simulink model "limbero_leg_control_DH"  (R2022a)
settings: Solver=ode45  StartTime=0.0  StopTime=8.00  RelTol=1e-3
undefined symbols (not defined in the file): a, a_contact, alpha, alpha_contact, d, d_contact, kpp, kpv, L, masses, masses_contact, offset, offset_contact, q_dotdot, qz, r_cm, r_cm_contact, t0, t_acc, T_lpf, t_tot, T_vel, Tc, Tiv
libraries: roblocks x4
settings Model: Creator=rubbe  LastModifiedBy=ale
settings ModelReferenceCC: EnableRefExpFcnMdlSchedulingChecks=off
settings RTWCC: Description=Generic Real-Time Target

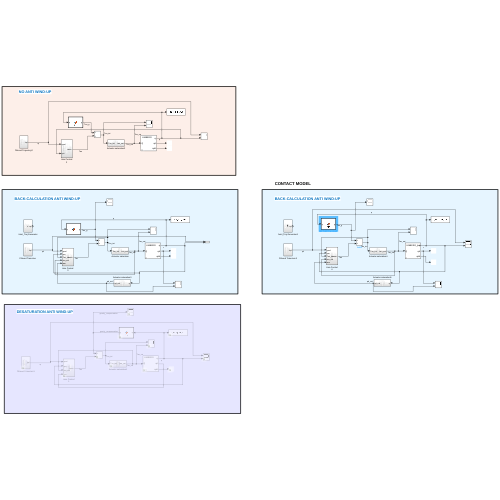
[thumbnail: Simulink's stored preview of the top-level diagram]
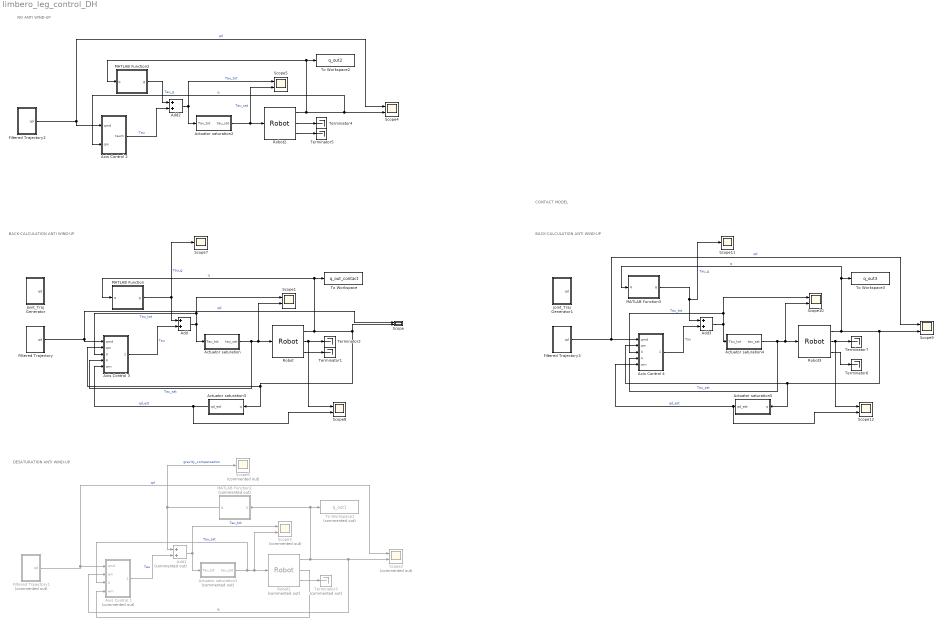
== system limbero_leg_control_DH ==
  note: CONTACT MODEL
  note: NO ANTI WIND-UP
  note: BACK-CALCULATION ANTI WIND-UP
  note: DESATURATION ANTI WIND-UP
  note: BACK-CALCULATION ANTI WIND-UP
  Actuator saturation : Subsystem
  Actuator saturation1 : Subsystem  Commented=on
  Actuator saturation2 : Subsystem
  Actuator saturation3 : Subsystem
  Actuator saturation4 : Subsystem
  Actuator saturation5 : Subsystem
  Add : Sum
  Add1 : Sum  Commented=on
  Add2 : Sum
  Add3 : Sum
  Axis Control 1 : Subsystem  Commented=on
  Axis Control 2 : Subsystem
  Axis Control 3 : Subsystem
  Axis Control 4 : Subsystem
  Filtered Trajectory : Subsystem
  Filtered Trajectory1 : Subsystem  Commented=on
  Filtered Trajectory2 : Subsystem
  Filtered Trajectory3 : Subsystem
  Joint_Traj Generator : Subsystem
  Joint_Traj Generator1 : Subsystem
  MATLAB Function : MATLAB Function  TreatAsAtomicUnit=on
  MATLAB Function1 : MATLAB Function  Commented=on  TreatAsAtomicUnit=on
  MATLAB Function2 : MATLAB Function  TreatAsAtomicUnit=on
  MATLAB Function3 : MATLAB Function  TreatAsAtomicUnit=on
  Robot : roblocks/Arm/Robot  robot=limbero  q0=qz'
  Robot1 : roblocks/Arm/Robot  Commented=on  robot=limbero  q0=qz'
  Robot2 : roblocks/Arm/Robot  robot=limbero  q0=qz'
  Robot3 : roblocks/Arm/Robot  robot=limbero_contact  q0=qz'
  Scope{,1,4..5,8..10,12} (8 alike) : Scope  NumInputPorts=2
  Scope11 : Scope
  Scope2 : Scope  Commented=on  NumInputPorts=2
  Scope3 : Scope  Commented=on  NumInputPorts=2
  Scope6 : Scope  Commented=on
  Scope7 : Scope
  Terminator{1..2,4..7} (6 alike) : Terminator
  Terminator3 : Terminator  Commented=on
  To Workspace : ToWorkspace  VariableName=q_out_contact  SaveFormat=Timeseries  SampleTime=-1
  To Workspace1 : ToWorkspace  Commented=on  VariableName=q_out1  SaveFormat=Timeseries  SampleTime=-1
  To Workspace2 : ToWorkspace  VariableName=q_out2  SaveFormat=Timeseries  SampleTime=-1
  To Workspace3 : ToWorkspace  VariableName=q_out3  SaveFormat=Timeseries  SampleTime=-1
  wires:
  Robot/3 -> Terminator1/1
  Robot/1 -> MATLAB Function/1(q), To Workspace/1, Axis Control 3/2(qm), Actuator saturation3/1(q), Scope/2  "q"
  MATLAB Function/1(g) -> Add/1, Scope7/1  "Tau_g"
  Filtered Trajectory/1(qd) -> Axis Control 3/1(qmd), Scope/1  "qd"
  Add/1 -> Axis Control 3/3(Tau_tot), Scope1/1, Actuator saturation/1(Tau_tot)  "Tau_tot"
  Actuator saturation/1(tau_sat) -> Axis Control 3/4(tau_sat), Robot/1, Scope1/2  "Tau_sat"
  Filtered Trajectory1/1(qd) -> Scope2/1, Axis Control 1/1(qmd)  "qd"
  Axis Control 1/1("taum ") -> Add1/2  "Tau"
  Actuator saturation1/1(tau_sat) -> Axis Control 1/3(tau_sat), Robot1/1, Scope3/2  "Tau_sat"
  Add1/1 -> Scope3/1, Actuator saturation1/1(Tau_tot)  "Tau_tot"
  Robot1/1 -> To Workspace1/1, MATLAB Function1/1(q), Scope2/2, Axis Control 1/2(qm)  "q"
  Robot1/3 -> Terminator3/1
  MATLAB Function1/1(g) -> Scope6/1, Add1/1  "gravity_compensation"
  Robot1/2 -> Axis Control 1/4(wm)
  Filtered Trajectory2/1(qd) -> Scope4/1, Axis Control 2/1(qmd)  "qd"
  Axis Control 2/1("taum ") -> Add2/2  "Tau"
  Actuator saturation2/1(tau_sat) -> Robot2/1, Scope5/2  "Tau_sat"
  Add2/1 -> Scope5/1, Actuator saturation2/1(Tau_tot)  "Tau_tot"
  Robot2/1 -> MATLAB Function2/1(q), To Workspace2/1, Scope4/2, Axis Control 2/2(qm)  "q"
  Robot2/3 -> Terminator5/1
  MATLAB Function2/1(g) -> Add2/1  "Tau_g"
  Robot2/2 -> Terminator4/1
  Axis Control 3/1("taum ") -> Add/2  "Tau"
  Robot/2 -> Scope8/1, Terminator2/1
  Actuator saturation3/1(qd_est) -> Scope8/2, Axis Control 3/5(wm)  "qd_est"
  Add3/1 -> Axis Control 4/3(Tau_tot), Scope10/1, Actuator saturation4/1(Tau_tot)  "Tau_tot"
  Filtered Trajectory3/1(qd) -> Axis Control 4/1(qmd), Scope9/1  "qd"
  Robot3/1 -> MATLAB Function3/1(q), To Workspace3/1, Axis Control 4/2(qm), Actuator saturation5/1(q), Scope9/2  "q"
  MATLAB Function3/1(g) -> Scope11/1, Add3/1  "Tau_g"
  Robot3/3 -> Terminator6/1
  Robot3/2 -> Scope12/1, Terminator7/1
  Actuator saturation4/1(tau_sat) -> Axis Control 4/4(tau_sat), Robot3/1, Scope10/2  "Tau_sat"
  Actuator saturation5/1(qd_est) -> Scope12/2, Axis Control 4/5(wm)  "qd_est"
  Axis Control 4/1("taum ") -> Add3/2  "Tau"

== system limbero_leg_control_DH/Actuator saturation ==
  Tau_tot : Inport
  Demux : Demux  Outputs=7
  Mux : Mux  Inputs=7
  Saturation : Saturate  UpperLimit=20.0  LowerLimit=-20.0
  Saturation1 : Saturate  UpperLimit=20.0  LowerLimit=-20.0
  Saturation2 : Saturate  UpperLimit=12.0  LowerLimit=-12.0
  Saturation3 : Saturate  UpperLimit=14.0  LowerLimit=-14.0
  Saturation4 : Saturate  UpperLimit=12.0  LowerLimit=-12.0
  Saturation5 : Saturate  UpperLimit=14.0  LowerLimit=-14.0
  Saturation6 : Saturate  UpperLimit=12.0  LowerLimit=-12.0
  tau_sat : Outport
  wires:
  Saturation6/1 -> Mux/7
  Mux/1 -> tau_sat/1
  Saturation3/1 -> Mux/4
  Tau_tot/1 -> Demux/1
  Demux/4 -> Saturation3/1
  Demux/7 -> Saturation6/1
  Saturation4/1 -> Mux/5
  Saturation1/1 -> Mux/2
  Demux/3 -> Saturation2/1
  Demux/1 -> Saturation/1
  Demux/5 -> Saturation4/1
  Demux/6 -> Saturation5/1
  Demux/2 -> Saturation1/1
  Saturation/1 -> Mux/1
  Saturation5/1 -> Mux/6
  Saturation2/1 -> Mux/3

== system limbero_leg_control_DH/Actuator saturation1 ==
  Tau_tot : Inport
  Demux : Demux  Outputs=7
  Mux : Mux  Inputs=7
  Saturation : Saturate  UpperLimit=20.0  LowerLimit=-20.0
  Saturation1 : Saturate  UpperLimit=20.0  LowerLimit=-20.0
  Saturation2 : Saturate  UpperLimit=12.0  LowerLimit=-12.0
  Saturation3 : Saturate  UpperLimit=14.0  LowerLimit=-14.0
  Saturation4 : Saturate  UpperLimit=12.0  LowerLimit=-12.0
  Saturation5 : Saturate  UpperLimit=14.0  LowerLimit=-14.0
  Saturation6 : Saturate  UpperLimit=12.0  LowerLimit=-12.0
  tau_sat : Outport
  wires:
  Saturation6/1 -> Mux/7
  Mux/1 -> tau_sat/1
  Saturation3/1 -> Mux/4
  Tau_tot/1 -> Demux/1
  Demux/4 -> Saturation3/1
  Demux/7 -> Saturation6/1
  Saturation4/1 -> Mux/5
  Saturation1/1 -> Mux/2
  Demux/3 -> Saturation2/1
  Demux/1 -> Saturation/1
  Demux/5 -> Saturation4/1
  Demux/6 -> Saturation5/1
  Demux/2 -> Saturation1/1
  Saturation/1 -> Mux/1
  Saturation5/1 -> Mux/6
  Saturation2/1 -> Mux/3

== system limbero_leg_control_DH/Actuator saturation2 ==
  Tau_tot : Inport
  Demux : Demux  Outputs=7
  Mux : Mux  Inputs=7
  Saturation : Saturate  UpperLimit=20.0  LowerLimit=-20.0
  Saturation1 : Saturate  UpperLimit=20.0  LowerLimit=-20.0
  Saturation2 : Saturate  UpperLimit=12.0  LowerLimit=-12.0
  Saturation3 : Saturate  UpperLimit=14.0  LowerLimit=-14.0
  Saturation4 : Saturate  UpperLimit=12.0  LowerLimit=-12.0
  Saturation5 : Saturate  UpperLimit=14.0  LowerLimit=-14.0
  Saturation6 : Saturate  UpperLimit=12.0  LowerLimit=-12.0
  tau_sat : Outport
  wires:
  Saturation6/1 -> Mux/7
  Mux/1 -> tau_sat/1
  Saturation3/1 -> Mux/4
  Tau_tot/1 -> Demux/1
  Demux/4 -> Saturation3/1
  Demux/7 -> Saturation6/1
  Saturation4/1 -> Mux/5
  Saturation1/1 -> Mux/2
  Demux/3 -> Saturation2/1
  Demux/1 -> Saturation/1
  Demux/5 -> Saturation4/1
  Demux/6 -> Saturation5/1
  Demux/2 -> Saturation1/1
  Saturation/1 -> Mux/1
  Saturation5/1 -> Mux/6
  Saturation2/1 -> Mux/3

== system limbero_leg_control_DH/Actuator saturation3 ==
  q : Inport
  Demux : Demux  Outputs=7
  Mux : Mux  Inputs=7
  Transfer Fcn{,1..6} (7 alike) : TransferFcn  Numerator=[1 0]  Denominator=[T_vel 1]
  qd_est : Outport
  wires:
  Mux/1 -> qd_est/1
  q/1 -> Demux/1
  Demux/4 -> Transfer Fcn3/1
  Demux/7 -> Transfer Fcn6/1
  Transfer Fcn1/1 -> Mux/2
  Demux/3 -> Transfer Fcn2/1
  Demux/1 -> Transfer Fcn/1
  Demux/5 -> Transfer Fcn4/1
  Demux/6 -> Transfer Fcn5/1
  Demux/2 -> Transfer Fcn1/1
  Transfer Fcn/1 -> Mux/1
  Transfer Fcn6/1 -> Mux/7
  Transfer Fcn5/1 -> Mux/6
  Transfer Fcn4/1 -> Mux/5
  Transfer Fcn3/1 -> Mux/4
  Transfer Fcn2/1 -> Mux/3

== system limbero_leg_control_DH/Actuator saturation4 ==
  Tau_tot : Inport
  Demux : Demux  Outputs=7
  Mux : Mux  Inputs=7
  Saturation : Saturate  UpperLimit=20.0  LowerLimit=-20.0
  Saturation1 : Saturate  UpperLimit=20.0  LowerLimit=-20.0
  Saturation2 : Saturate  UpperLimit=12.0  LowerLimit=-12.0
  Saturation3 : Saturate  UpperLimit=14.0  LowerLimit=-14.0
  Saturation4 : Saturate  UpperLimit=12.0  LowerLimit=-12.0
  Saturation5 : Saturate  UpperLimit=14.0  LowerLimit=-14.0
  Saturation6 : Saturate  UpperLimit=12.0  LowerLimit=-12.0
  tau_sat : Outport
  wires:
  Saturation6/1 -> Mux/7
  Mux/1 -> tau_sat/1
  Saturation3/1 -> Mux/4
  Tau_tot/1 -> Demux/1
  Demux/4 -> Saturation3/1
  Demux/7 -> Saturation6/1
  Saturation4/1 -> Mux/5
  Saturation1/1 -> Mux/2
  Demux/3 -> Saturation2/1
  Demux/1 -> Saturation/1
  Demux/5 -> Saturation4/1
  Demux/6 -> Saturation5/1
  Demux/2 -> Saturation1/1
  Saturation/1 -> Mux/1
  Saturation5/1 -> Mux/6
  Saturation2/1 -> Mux/3

== system limbero_leg_control_DH/Actuator saturation5 ==
  q : Inport
  Demux : Demux  Outputs=7
  Mux : Mux  Inputs=7
  Transfer Fcn{,1..6} (7 alike) : TransferFcn  Numerator=[1 0]  Denominator=[T_vel 1]
  qd_est : Outport
  wires:
  Mux/1 -> qd_est/1
  q/1 -> Demux/1
  Demux/4 -> Transfer Fcn3/1
  Demux/7 -> Transfer Fcn6/1
  Transfer Fcn1/1 -> Mux/2
  Demux/3 -> Transfer Fcn2/1
  Demux/1 -> Transfer Fcn/1
  Demux/5 -> Transfer Fcn4/1
  Demux/6 -> Transfer Fcn5/1
  Demux/2 -> Transfer Fcn1/1
  Transfer Fcn/1 -> Mux/1
  Transfer Fcn6/1 -> Mux/7
  Transfer Fcn5/1 -> Mux/6
  Transfer Fcn4/1 -> Mux/5
  Transfer Fcn3/1 -> Mux/4
  Transfer Fcn2/1 -> Mux/3

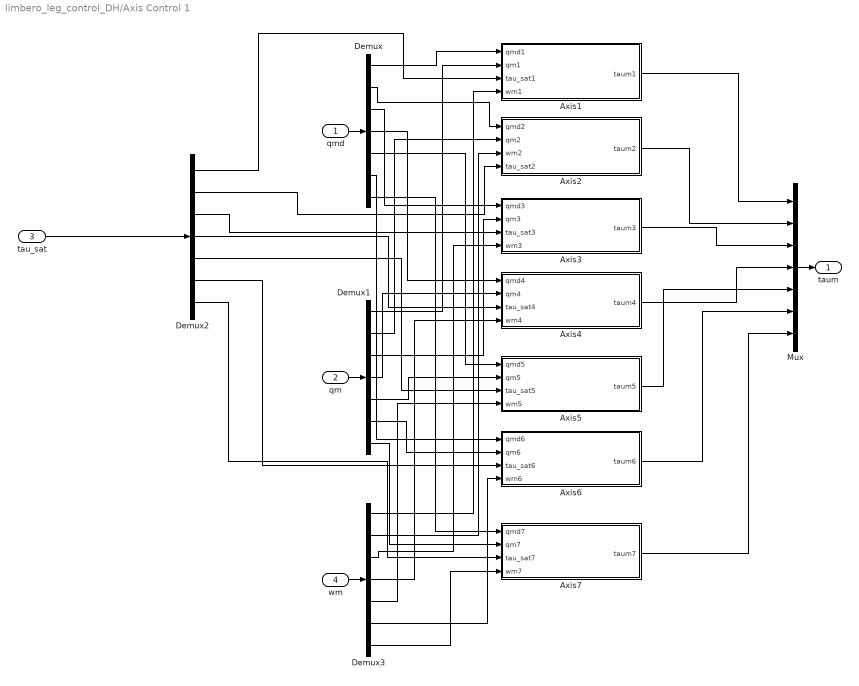
== system limbero_leg_control_DH/Axis Control 1 ==
  qmd : Inport
  qm : Inport  Port=2
  tau_sat : Inport  Port=3
  wm : Inport  Port=4
  "Axis1 " : Subsystem
  "Axis2 " : Subsystem
  "Axis3 " : Subsystem
  "Axis4 " : Subsystem
  "Axis5 " : Subsystem
  "Axis6 " : Subsystem
  "Axis7 " : Subsystem
  Demux{,1..3} (4 alike) : Demux  Outputs=7
  Mux : Mux  Inputs=7
  "taum " : Outport  VectorParamsAs1DForOutWhenUnconnected=off
  wires:
  "Axis5 "/1(taum5) -> Mux/5
  Demux1/1 -> "Axis1 "/2(qm1)
  Demux1/3 -> "Axis3 "/2(qm3)
  Demux/1 -> "Axis1 "/1(qmd1)
  "Axis4 "/1(taum4) -> Mux/4
  "Axis3 "/1(taum3) -> Mux/3
  "Axis6 "/1(taum6) -> Mux/6
  "Axis1 "/1(taum1) -> Mux/1
  Mux/1 -> "taum "/1
  Demux/2 -> "Axis2 "/1(qmd2)
  Demux/4 -> "Axis4 "/1(qmd4)
  Demux/3 -> "Axis3 "/1(qmd3)
  Demux/6 -> "Axis6 "/1(qmd6)
  Demux/5 -> "Axis5 "/1(qmd5)
  Demux1/4 -> "Axis4 "/2(qm4)
  Demux1/6 -> "Axis6 "/2(qm6)
  Demux1/5 -> "Axis5 "/2(qm5)
  Demux1/2 -> "Axis2 "/2(qm2)
  qm/1 -> Demux1/1
  qmd/1 -> Demux/1
  Demux1/7 -> "Axis7 "/2(qm7)
  Demux/7 -> "Axis7 "/1(qmd7)
  "Axis7 "/1(taum7) -> Mux/7
  Demux2/7 -> "Axis7 "/3(tau_sat7)
  tau_sat/1 -> Demux2/1
  Demux2/6 -> "Axis6 "/3(tau_sat6)
  Demux2/5 -> "Axis5 "/3(tau_sat5)
  Demux2/4 -> "Axis4 "/3(tau_sat4)
  Demux2/3 -> "Axis3 "/3(tau_sat3)
  Demux2/1 -> "Axis1 "/3(tau_sat1)
  wm/1 -> Demux3/1
  Demux3/1 -> "Axis1 "/4(wm1)
  Demux3/2 -> "Axis2 "/3(wm2)
  Demux3/3 -> "Axis3 "/4(wm3)
  Demux3/4 -> "Axis4 "/4(wm4)
  Demux3/5 -> "Axis5 "/4(wm5)
  Demux3/6 -> "Axis6 "/4(wm6)
  Demux3/7 -> "Axis7 "/4(wm7)
  Demux2/2 -> "Axis2 "/4(tau_sat2)
  "Axis2 "/1(taum2) -> Mux/2

== system limbero_leg_control_DH/Axis Control 2 ==
  qmd : Inport
  qm : Inport  Port=2
  "Axis1 " : Subsystem
  "Axis2 " : Subsystem
  "Axis3 " : Subsystem
  "Axis4 " : Subsystem
  "Axis5 " : Subsystem
  "Axis6 " : Subsystem
  "Axis7 " : Subsystem
  Demux : Demux  Outputs=7
  Demux1 : Demux  Outputs=7
  Mux : Mux  Inputs=7
  "taum " : Outport  VectorParamsAs1DForOutWhenUnconnected=off
  wires:
  "Axis5 "/1(taum5) -> Mux/5
  Demux1/1 -> "Axis1 "/2(qm1)
  "Axis2 "/1(taum2) -> Mux/2
  Demux1/3 -> "Axis3 "/2(qm3)
  Demux/1 -> "Axis1 "/1(qmd1)
  "Axis4 "/1(taum4) -> Mux/4
  "Axis3 "/1(taum3) -> Mux/3
  "Axis6 "/1(taum6) -> Mux/6
  "Axis1 "/1(taum1) -> Mux/1
  Mux/1 -> "taum "/1
  Demux/2 -> "Axis2 "/1(qmd2)
  Demux/4 -> "Axis4 "/1(qmd4)
  Demux/3 -> "Axis3 "/1(qmd3)
  Demux/6 -> "Axis6 "/1(qmd6)
  Demux/5 -> "Axis5 "/1(qmd5)
  Demux1/4 -> "Axis4 "/2(qm4)
  Demux1/6 -> "Axis6 "/2(qm6)
  Demux1/5 -> "Axis5 "/2(qm5)
  Demux1/2 -> "Axis2 "/2(qm2)
  qm/1 -> Demux1/1
  qmd/1 -> Demux/1
  Demux1/7 -> "Axis7 "/2(qm7)
  Demux/7 -> "Axis7 "/1(qmd7)
  "Axis7 "/1(taum7) -> Mux/7

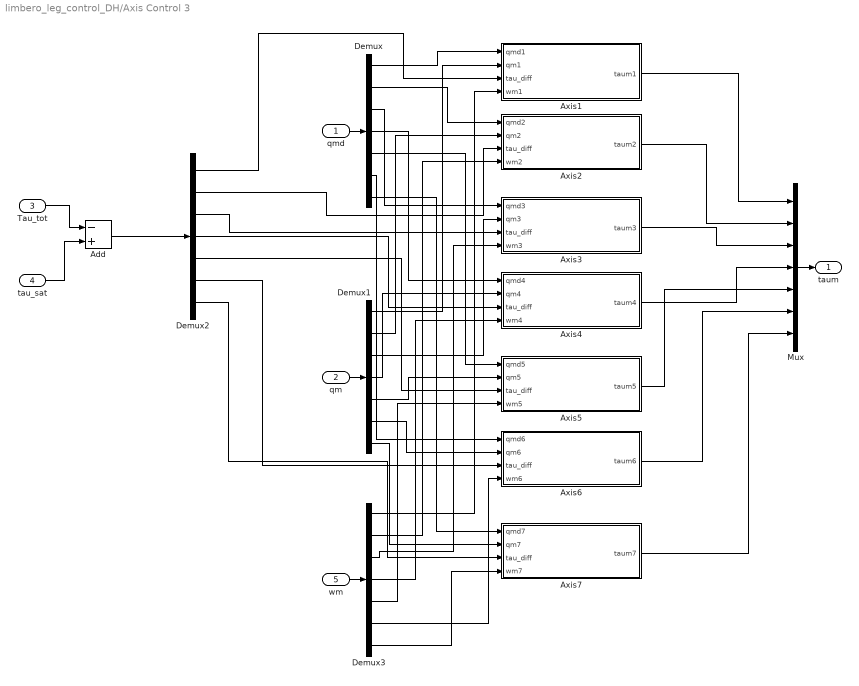
== system limbero_leg_control_DH/Axis Control 3 ==
  qmd : Inport
  qm : Inport  Port=2
  Tau_tot : Inport  Port=3
  tau_sat : Inport  Port=4
  wm : Inport  Port=5
  Add : Sum  Inputs=-+
  "Axis1 " : Subsystem
  "Axis2 " : Subsystem
  "Axis3 " : Subsystem
  "Axis4 " : Subsystem
  "Axis5 " : Subsystem
  "Axis6 " : Subsystem
  "Axis7 " : Subsystem
  Demux{,1..3} (4 alike) : Demux  Outputs=7
  Mux : Mux  Inputs=7
  "taum " : Outport  VectorParamsAs1DForOutWhenUnconnected=off
  wires:
  "Axis5 "/1(taum5) -> Mux/5
  Demux1/1 -> "Axis1 "/2(qm1)
  "Axis2 "/1(taum2) -> Mux/2
  Demux1/3 -> "Axis3 "/2(qm3)
  Demux/1 -> "Axis1 "/1(qmd1)
  "Axis4 "/1(taum4) -> Mux/4
  "Axis3 "/1(taum3) -> Mux/3
  "Axis6 "/1(taum6) -> Mux/6
  "Axis1 "/1(taum1) -> Mux/1
  Mux/1 -> "taum "/1
  Demux/2 -> "Axis2 "/1(qmd2)
  Demux/4 -> "Axis4 "/1(qmd4)
  Demux/3 -> "Axis3 "/1(qmd3)
  Demux/6 -> "Axis6 "/1(qmd6)
  Demux/5 -> "Axis5 "/1(qmd5)
  Demux1/4 -> "Axis4 "/2(qm4)
  Demux1/6 -> "Axis6 "/2(qm6)
  Demux1/5 -> "Axis5 "/2(qm5)
  Demux1/2 -> "Axis2 "/2(qm2)
  qm/1 -> Demux1/1
  qmd/1 -> Demux/1
  Demux1/7 -> "Axis7 "/2(qm7)
  Demux/7 -> "Axis7 "/1(qmd7)
  "Axis7 "/1(taum7) -> Mux/7
  Tau_tot/1 -> Add/1
  tau_sat/1 -> Add/2
  Demux2/7 -> "Axis7 "/3(tau_diff)
  Add/1 -> Demux2/1
  Demux2/6 -> "Axis6 "/3(tau_diff)
  Demux2/5 -> "Axis5 "/3(tau_diff)
  Demux2/4 -> "Axis4 "/3(tau_diff)
  Demux2/3 -> "Axis3 "/3(tau_diff)
  Demux2/2 -> "Axis2 "/3(tau_diff)
  Demux2/1 -> "Axis1 "/3(tau_diff)
  wm/1 -> Demux3/1
  Demux3/1 -> "Axis1 "/4(wm1)
  Demux3/2 -> "Axis2 "/4(wm2)
  Demux3/3 -> "Axis3 "/4(wm3)
  Demux3/4 -> "Axis4 "/4(wm4)
  Demux3/5 -> "Axis5 "/4(wm5)
  Demux3/6 -> "Axis6 "/4(wm6)
  Demux3/7 -> "Axis7 "/4(wm7)

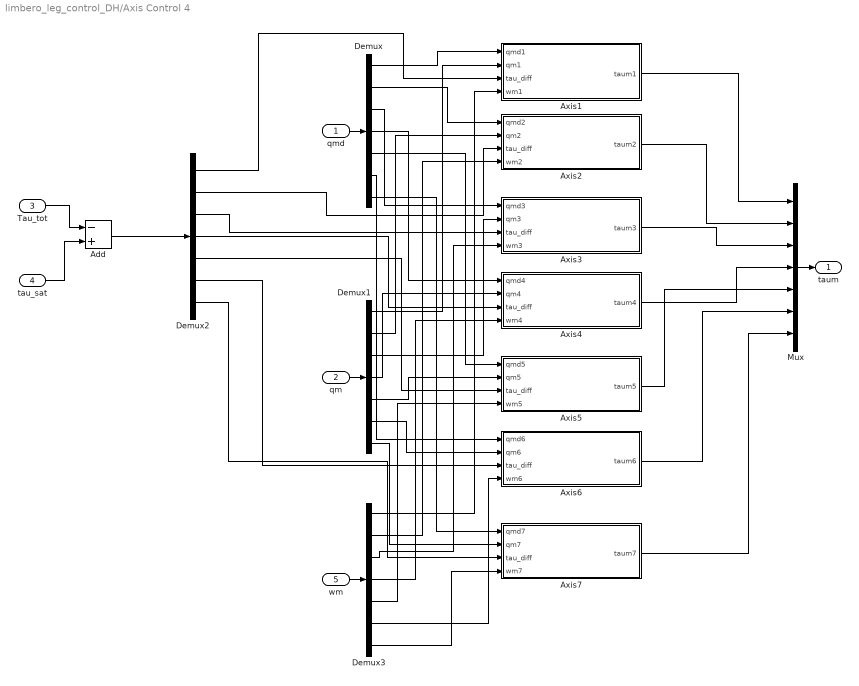
== system limbero_leg_control_DH/Axis Control 4 ==
  qmd : Inport
  qm : Inport  Port=2
  Tau_tot : Inport  Port=3
  tau_sat : Inport  Port=4
  wm : Inport  Port=5
  Add : Sum  Inputs=-+
  "Axis1 " : Subsystem
  "Axis2 " : Subsystem
  "Axis3 " : Subsystem
  "Axis4 " : Subsystem
  "Axis5 " : Subsystem
  "Axis6 " : Subsystem
  "Axis7 " : Subsystem
  Demux{,1..3} (4 alike) : Demux  Outputs=7
  Mux : Mux  Inputs=7
  "taum " : Outport  VectorParamsAs1DForOutWhenUnconnected=off
  wires:
  "Axis5 "/1(taum5) -> Mux/5
  Demux1/1 -> "Axis1 "/2(qm1)
  "Axis2 "/1(taum2) -> Mux/2
  Demux1/3 -> "Axis3 "/2(qm3)
  Demux/1 -> "Axis1 "/1(qmd1)
  "Axis4 "/1(taum4) -> Mux/4
  "Axis3 "/1(taum3) -> Mux/3
  "Axis6 "/1(taum6) -> Mux/6
  "Axis1 "/1(taum1) -> Mux/1
  Mux/1 -> "taum "/1
  Demux/2 -> "Axis2 "/1(qmd2)
  Demux/4 -> "Axis4 "/1(qmd4)
  Demux/3 -> "Axis3 "/1(qmd3)
  Demux/6 -> "Axis6 "/1(qmd6)
  Demux/5 -> "Axis5 "/1(qmd5)
  Demux1/4 -> "Axis4 "/2(qm4)
  Demux1/6 -> "Axis6 "/2(qm6)
  Demux1/5 -> "Axis5 "/2(qm5)
  Demux1/2 -> "Axis2 "/2(qm2)
  qm/1 -> Demux1/1
  qmd/1 -> Demux/1
  Demux1/7 -> "Axis7 "/2(qm7)
  Demux/7 -> "Axis7 "/1(qmd7)
  "Axis7 "/1(taum7) -> Mux/7
  Tau_tot/1 -> Add/1
  tau_sat/1 -> Add/2
  Demux2/7 -> "Axis7 "/3(tau_diff)
  Add/1 -> Demux2/1
  Demux2/6 -> "Axis6 "/3(tau_diff)
  Demux2/5 -> "Axis5 "/3(tau_diff)
  Demux2/4 -> "Axis4 "/3(tau_diff)
  Demux2/3 -> "Axis3 "/3(tau_diff)
  Demux2/2 -> "Axis2 "/3(tau_diff)
  Demux2/1 -> "Axis1 "/3(tau_diff)
  wm/1 -> Demux3/1
  Demux3/1 -> "Axis1 "/4(wm1)
  Demux3/2 -> "Axis2 "/4(wm2)
  Demux3/3 -> "Axis3 "/4(wm3)
  Demux3/4 -> "Axis4 "/4(wm4)
  Demux3/5 -> "Axis5 "/4(wm5)
  Demux3/6 -> "Axis6 "/4(wm6)
  Demux3/7 -> "Axis7 "/4(wm7)

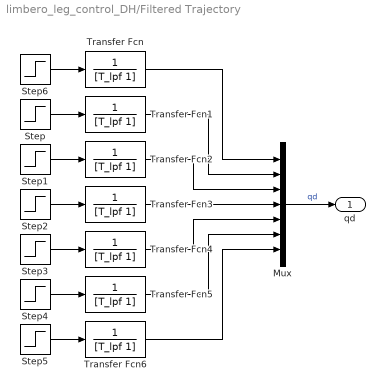
== system limbero_leg_control_DH/Filtered Trajectory ==
  Mux : Mux  Inputs=7
  Step{,1..2,5..6} (5 alike) : Step  Time=0  After=0  SampleTime=0
  Step3 : Step  After=-pi/6  SampleTime=0
  Step4 : Step  Time=2  After=-pi/8  SampleTime=0
  Transfer Fcn{,1..6} (7 alike) : TransferFcn  Denominator=[T_lpf 1]
  qd : Outport
  wires:
  Step3/1 -> Transfer Fcn4/1
  Step1/1 -> Transfer Fcn2/1
  Step4/1 -> Transfer Fcn5/1
  Transfer Fcn/1 -> Mux/1
  Transfer Fcn6/1 -> Mux/7
  Transfer Fcn3/1 -> Mux/4
  Transfer Fcn5/1 -> Mux/6
  Step2/1 -> Transfer Fcn3/1
  Step/1 -> Transfer Fcn1/1
  Step6/1 -> Transfer Fcn/1
  Transfer Fcn2/1 -> Mux/3
  Transfer Fcn4/1 -> Mux/5
  Transfer Fcn1/1 -> Mux/2
  Mux/1 -> qd/1  "qd"
  Step5/1 -> Transfer Fcn6/1

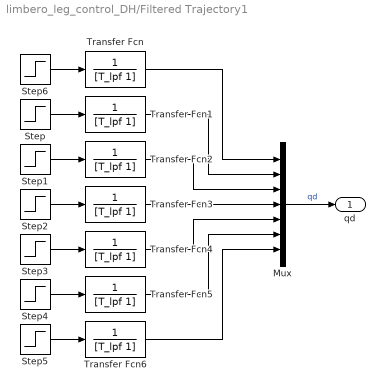
== system limbero_leg_control_DH/Filtered Trajectory1 ==
  Mux : Mux  Inputs=7
  Step : Step  After=-pi/6  SampleTime=0
  Step1 : Step  After=pi/2  SampleTime=0
  Step2 : Step  After=0  SampleTime=0
  Step3 : Step  Time=0  After=0  SampleTime=0
  Step4 : Step  Time=0  After=0  SampleTime=0
  Step5 : Step  Time=0  After=0  SampleTime=0
  Step6 : Step  Time=0.5  After=pi/4  SampleTime=0
  Transfer Fcn{,1..6} (7 alike) : TransferFcn  Denominator=[T_lpf 1]
  qd : Outport
  wires:
  Step3/1 -> Transfer Fcn4/1
  Step1/1 -> Transfer Fcn2/1
  Step4/1 -> Transfer Fcn5/1
  Transfer Fcn/1 -> Mux/1
  Transfer Fcn6/1 -> Mux/7
  Transfer Fcn3/1 -> Mux/4
  Transfer Fcn5/1 -> Mux/6
  Step2/1 -> Transfer Fcn3/1
  Step/1 -> Transfer Fcn1/1
  Step6/1 -> Transfer Fcn/1
  Transfer Fcn2/1 -> Mux/3
  Transfer Fcn4/1 -> Mux/5
  Transfer Fcn1/1 -> Mux/2
  Mux/1 -> qd/1  "qd"
  Step5/1 -> Transfer Fcn6/1

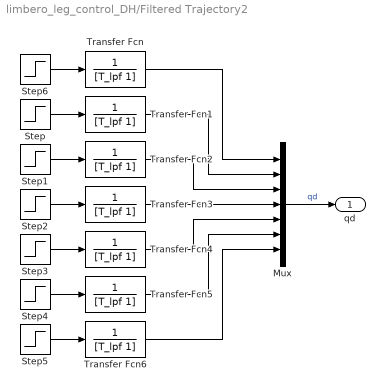
== system limbero_leg_control_DH/Filtered Trajectory2 ==
  Mux : Mux  Inputs=7
  Step : Step  After=-pi/6  SampleTime=0
  Step1 : Step  After=pi/2  SampleTime=0
  Step2 : Step  After=0  SampleTime=0
  Step3 : Step  Time=0  After=0  SampleTime=0
  Step4 : Step  Time=0  After=0  SampleTime=0
  Step5 : Step  Time=0  After=0  SampleTime=0
  Step6 : Step  Time=0.5  After=pi/4  SampleTime=0
  Transfer Fcn{,1..6} (7 alike) : TransferFcn  Denominator=[T_lpf 1]
  qd : Outport
  wires:
  Step3/1 -> Transfer Fcn4/1
  Step1/1 -> Transfer Fcn2/1
  Step4/1 -> Transfer Fcn5/1
  Transfer Fcn/1 -> Mux/1
  Transfer Fcn6/1 -> Mux/7
  Transfer Fcn3/1 -> Mux/4
  Transfer Fcn5/1 -> Mux/6
  Step2/1 -> Transfer Fcn3/1
  Step/1 -> Transfer Fcn1/1
  Step6/1 -> Transfer Fcn/1
  Transfer Fcn2/1 -> Mux/3
  Transfer Fcn4/1 -> Mux/5
  Transfer Fcn1/1 -> Mux/2
  Mux/1 -> qd/1  "qd"
  Step5/1 -> Transfer Fcn6/1

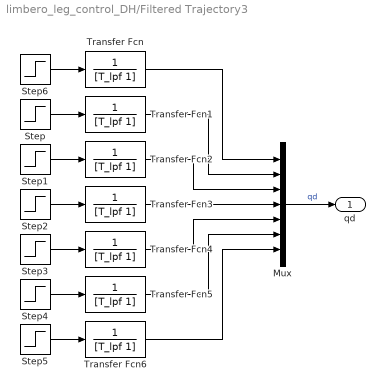
== system limbero_leg_control_DH/Filtered Trajectory3 ==
  Mux : Mux  Inputs=7
  Step : Step  After=-pi/6  SampleTime=0
  Step1 : Step  After=pi/2  SampleTime=0
  Step2 : Step  After=0  SampleTime=0
  Step3 : Step  Time=0  After=0  SampleTime=0
  Step4 : Step  Time=0  After=0  SampleTime=0
  Step5 : Step  Time=0  After=0  SampleTime=0
  Step6 : Step  Time=0.5  After=pi/4  SampleTime=0
  Transfer Fcn{,1..6} (7 alike) : TransferFcn  Denominator=[T_lpf 1]
  qd : Outport
  wires:
  Step3/1 -> Transfer Fcn4/1
  Step1/1 -> Transfer Fcn2/1
  Step4/1 -> Transfer Fcn5/1
  Transfer Fcn/1 -> Mux/1
  Transfer Fcn6/1 -> Mux/7
  Transfer Fcn3/1 -> Mux/4
  Transfer Fcn5/1 -> Mux/6
  Step2/1 -> Transfer Fcn3/1
  Step/1 -> Transfer Fcn1/1
  Step6/1 -> Transfer Fcn/1
  Transfer Fcn2/1 -> Mux/3
  Transfer Fcn4/1 -> Mux/5
  Transfer Fcn1/1 -> Mux/2
  Mux/1 -> qd/1  "qd"
  Step5/1 -> Transfer Fcn6/1

== system limbero_leg_control_DH/Joint_Traj Generator ==
  Constant : Constant  Value=0
  Mux : Mux  Inputs=7
  Subsystem : Subsystem
  Subsystem1 : Subsystem
  qd : Outport
  wires:
  Subsystem1/1(C2F) -> Mux/3
  Constant/1 -> Mux/7, Mux/6, Mux/5, Mux/4, Mux/1
  Subsystem/1(B2C) -> Mux/2
  Mux/1 -> qd/1

== system limbero_leg_control_DH/Joint_Traj Generator1 ==
  Constant : Constant  Value=0
  Mux : Mux  Inputs=7
  Subsystem : Subsystem
  Subsystem1 : Subsystem
  qd : Outport
  wires:
  Subsystem1/1(C2F) -> Mux/3
  Constant/1 -> Mux/7, Mux/6, Mux/5, Mux/4, Mux/1
  Subsystem/1(B2C) -> Mux/2
  Mux/1 -> qd/1

== system limbero_leg_control_DH/Axis Control 1/Axis1  ==
  qmd1 : Inport
  qm1 : Inport  Port=2
  tau_sat1 : Inport  Port=3
  wm1 : Inport  Port=4
  Add : Sum  Inputs=++-
  Add1 : Sum
  "Derivator qmd1 " : Derivative  CoefficientInTFapproximation=1/260
  Prop 1 : Gain  Gain=kpp
  Sum : Sum  Inputs=|+-
  Transfer Fcn4 : TransferFcn  Numerator=[kpv(1)*Tiv kpv(1)]  Denominator=[Tiv L]
  Transfer Fcn5 : TransferFcn  Numerator=[L]  Denominator=[Tiv L]
  taum1 : Outport  VectorParamsAs1DForOutWhenUnconnected=off
  wires:
  "Derivator qmd1 "/1 -> Add/1
  Sum/1 -> Prop 1/1
  qm1/1 -> Sum/2
  Prop 1/1 -> Add/2
  qmd1/1 -> "Derivator qmd1 "/1, Sum/1
  Add1/1 -> taum1/1
  wm1/1 -> Add/3  "wm1"
  Add/1 -> Transfer Fcn4/1
  Transfer Fcn4/1 -> Add1/1
  tau_sat1/1 -> Transfer Fcn5/1
  Transfer Fcn5/1 -> Add1/2  "anti_wind_up"

== system limbero_leg_control_DH/Axis Control 1/Axis2  ==
  qmd2 : Inport
  qm2 : Inport  Port=2
  wm2 : Inport  Port=3
  tau_sat2 : Inport  Port=4
  Add : Sum  Inputs=++-
  Add1 : Sum
  Derivator qmd2 : Derivative  CoefficientInTFapproximation=1/260
  Prop 2 : Gain  Gain=kpp
  Scope : Scope
  Scope1 : Scope
  Sum : Sum  Inputs=|+-
  Transfer Fcn4 : TransferFcn  Numerator=[kpv(2)*Tiv kpv(2)]  Denominator=[Tiv L]
  Transfer Fcn5 : TransferFcn  Numerator=[L]  Denominator=[Tiv L]
  taum2 : Outport  VectorParamsAs1DForOutWhenUnconnected=off
  wires:
  Derivator qmd2/1 -> Add/1
  Sum/1 -> Prop 2/1
  qm2/1 -> Sum/2
  Prop 2/1 -> Add/2
  qmd2/1 -> Derivator qmd2/1, Sum/1
  wm2/1 -> Add/3
  tau_sat2/1 -> Transfer Fcn5/1
  Transfer Fcn4/1 -> Add1/1
  Add/1 -> Scope/1, Transfer Fcn4/1  "e_w"
  Transfer Fcn5/1 -> Scope1/1, Add1/2  "anti_wind_up"
  Add1/1 -> taum2/1

== system limbero_leg_control_DH/Axis Control 1/Axis3  ==
  qmd3 : Inport
  qm3 : Inport  Port=2
  tau_sat3 : Inport  Port=3
  wm3 : Inport  Port=4
  Add : Sum  Inputs=++-
  Add1 : Sum
  Derivator qmd3 : Derivative  CoefficientInTFapproximation=1/260
  Prop 3 : Gain  Gain=kpp
  Sum : Sum  Inputs=|+-
  Transfer Fcn4 : TransferFcn  Numerator=[kpv(3)*Tiv kpv(3)]  Denominator=[Tiv L]
  Transfer Fcn5 : TransferFcn  Numerator=[L]  Denominator=[Tiv L]
  taum3 : Outport  VectorParamsAs1DForOutWhenUnconnected=off
  wires:
  Derivator qmd3/1 -> Add/1
  wm3/1 -> Add/3
  Sum/1 -> Prop 3/1
  qm3/1 -> Sum/2
  Prop 3/1 -> Add/2
  qmd3/1 -> Derivator qmd3/1, Sum/1
  Add1/1 -> taum3/1
  Transfer Fcn5/1 -> Add1/2  "anti_wind_up"
  Transfer Fcn4/1 -> Add1/1
  Add/1 -> Transfer Fcn4/1
  tau_sat3/1 -> Transfer Fcn5/1

== system limbero_leg_control_DH/Axis Control 1/Axis4  ==
  qmd4 : Inport
  qm4 : Inport  Port=2
  tau_sat4 : Inport  Port=3
  wm4 : Inport  Port=4
  Add : Sum  Inputs=++-
  Add1 : Sum
  Derivator qmd4 : Derivative  CoefficientInTFapproximation=1/700
  Prop 4 : Gain  Gain=kpp
  Sum : Sum  Inputs=|+-
  Transfer Fcn4 : TransferFcn  Numerator=[kpv(4)*Tiv kpv(4)]  Denominator=[Tiv L]
  Transfer Fcn5 : TransferFcn  Numerator=[L]  Denominator=[Tiv L]
  taum4 : Outport  VectorParamsAs1DForOutWhenUnconnected=off
  wires:
  Derivator qmd4/1 -> Add/1
  wm4/1 -> Add/3
  Sum/1 -> Prop 4/1
  qm4/1 -> Sum/2
  Prop 4/1 -> Add/2
  qmd4/1 -> Derivator qmd4/1, Sum/1
  tau_sat4/1 -> Transfer Fcn5/1
  Transfer Fcn5/1 -> Add1/2  "anti_wind_up"
  Transfer Fcn4/1 -> Add1/1
  Add/1 -> Transfer Fcn4/1
  Add1/1 -> taum4/1

== system limbero_leg_control_DH/Axis Control 1/Axis5  ==
  qmd5 : Inport
  qm5 : Inport  Port=2
  tau_sat5 : Inport  Port=3
  wm5 : Inport  Port=4
  Add : Sum  Inputs=++-
  Add1 : Sum
  Derivator qmd5 : Derivative  CoefficientInTFapproximation=1/700
  Prop 5 : Gain  Gain=kpp
  Sum : Sum  Inputs=|+-
  Transfer Fcn4 : TransferFcn  Numerator=[kpv(5)*Tiv kpv(5)]  Denominator=[Tiv L]
  Transfer Fcn5 : TransferFcn  Numerator=[L]  Denominator=[Tiv L]
  taum5 : Outport  VectorParamsAs1DForOutWhenUnconnected=off
  wires:
  Derivator qmd5/1 -> Add/1
  wm5/1 -> Add/3
  Sum/1 -> Prop 5/1
  qm5/1 -> Sum/2
  Prop 5/1 -> Add/2
  qmd5/1 -> Derivator qmd5/1, Sum/1
  tau_sat5/1 -> Transfer Fcn5/1
  Add1/1 -> taum5/1
  Transfer Fcn5/1 -> Add1/2  "anti_wind_up"
  Transfer Fcn4/1 -> Add1/1
  Add/1 -> Transfer Fcn4/1

== system limbero_leg_control_DH/Axis Control 1/Axis6  ==
  qmd6 : Inport
  qm6 : Inport  Port=2
  tau_sat6 : Inport  Port=3
  wm6 : Inport  Port=4
  Add : Sum  Inputs=++-
  Add1 : Sum
  Derivator qmd6 : Derivative  CoefficientInTFapproximation=1/700
  Prop 6 : Gain  Gain=kpp
  Sum : Sum  Inputs=|+-
  Transfer Fcn4 : TransferFcn  Numerator=[kpv(6)*Tiv kpv(6)]  Denominator=[Tiv L]
  Transfer Fcn5 : TransferFcn  Numerator=[L]  Denominator=[Tiv L]
  taum6 : Outport  VectorParamsAs1DForOutWhenUnconnected=off
  wires:
  Derivator qmd6/1 -> Add/1
  wm6/1 -> Add/3
  Sum/1 -> Prop 6/1
  qm6/1 -> Sum/2
  Prop 6/1 -> Add/2
  qmd6/1 -> Derivator qmd6/1, Sum/1
  Add1/1 -> taum6/1
  Transfer Fcn5/1 -> Add1/2  "anti_wind_up"
  Transfer Fcn4/1 -> Add1/1
  Add/1 -> Transfer Fcn4/1
  tau_sat6/1 -> Transfer Fcn5/1

== system limbero_leg_control_DH/Axis Control 1/Axis7  ==
  qmd7 : Inport
  qm7 : Inport  Port=2
  tau_sat7 : Inport  Port=3
  wm7 : Inport  Port=4
  Add : Sum  Inputs=++-
  Add1 : Sum
  Derivator qmd7 : Derivative  CoefficientInTFapproximation=1/700
  Prop 7 : Gain  Gain=kpp
  Sum : Sum  Inputs=|+-
  Transfer Fcn4 : TransferFcn  Numerator=[kpv(7)*Tiv kpv(7)]  Denominator=[Tiv L]
  Transfer Fcn5 : TransferFcn  Numerator=[L]  Denominator=[Tiv L]
  taum7 : Outport  VectorParamsAs1DForOutWhenUnconnected=off
  wires:
  qmd7/1 -> Sum/1, Derivator qmd7/1
  Prop 7/1 -> Add/2
  qm7/1 -> Sum/2
  Sum/1 -> Prop 7/1
  wm7/1 -> Add/3
  Derivator qmd7/1 -> Add/1
  tau_sat7/1 -> Transfer Fcn5/1
  Add1/1 -> taum7/1
  Transfer Fcn5/1 -> Add1/2  "anti_wind_up"
  Transfer Fcn4/1 -> Add1/1
  Add/1 -> Transfer Fcn4/1

== system limbero_leg_control_DH/Axis Control 2/Axis1  ==
  qmd1 : Inport
  qm1 : Inport  Port=2
  Add : Sum  Inputs=++-
  Add1 : Sum
  Gain : Gain  Gain=kpv(1)
  Gain1 : Gain  Gain=kpv(1)/Tiv
  Integrator : Integrator
  Prop 1 : Gain  Gain=kpp
  Sum : Sum  Inputs=|+-
  Transfer Fcn : TransferFcn  Numerator=[1 0]  Denominator=[T_vel 1]
  Transfer Fcn1 : TransferFcn  Numerator=[1 0]  Denominator=[T_vel 1]
  taum1 : Outport  VectorParamsAs1DForOutWhenUnconnected=off
  wires:
  Transfer Fcn1/1 -> Add/1
  Transfer Fcn/1 -> Add/3
  Sum/1 -> Prop 1/1
  qm1/1 -> Sum/2, Transfer Fcn/1
  Prop 1/1 -> Add/2
  Add/1 -> Gain1/1, Gain/1
  qmd1/1 -> Transfer Fcn1/1, Sum/1
  Add1/1 -> taum1/1
  Gain/1 -> Add1/1
  Integrator/1 -> Add1/2
  Gain1/1 -> Integrator/1

== system limbero_leg_control_DH/Axis Control 2/Axis2  ==
  qmd2 : Inport
  qm2 : Inport  Port=2
  Add : Sum  Inputs=++-
  Add1 : Sum
  Gain : Gain  Gain=kpv(2)
  Gain1 : Gain  Gain=kpv(2)/Tiv
  Integrator : Integrator
  Prop 2 : Gain  Gain=kpp
  Sum : Sum  Inputs=|+-
  Transfer Fcn : TransferFcn  Numerator=[1 0]  Denominator=[T_vel 1]
  Transfer Fcn1 : TransferFcn  Numerator=[1 0]  Denominator=[T_vel 1]
  taum2 : Outport  VectorParamsAs1DForOutWhenUnconnected=off
  wires:
  Transfer Fcn1/1 -> Add/1
  Transfer Fcn/1 -> Add/3
  Sum/1 -> Prop 2/1
  qm2/1 -> Transfer Fcn/1, Sum/2
  Prop 2/1 -> Add/2
  qmd2/1 -> Transfer Fcn1/1, Sum/1
  Gain1/1 -> Integrator/1
  Gain/1 -> Add1/1
  Add/1 -> Gain1/1, Gain/1
  Integrator/1 -> Add1/2
  Add1/1 -> taum2/1

== system limbero_leg_control_DH/Axis Control 2/Axis3  ==
  qmd3 : Inport
  qm3 : Inport  Port=2
  Add : Sum  Inputs=++-
  Add1 : Sum
  Gain : Gain  Gain=kpv(3)
  Gain1 : Gain  Gain=kpv(3)/Tiv
  Integrator : Integrator
  Prop 3 : Gain  Gain=kpp
  Sum : Sum  Inputs=|+-
  Transfer Fcn : TransferFcn  Numerator=[1 0]  Denominator=[T_vel 1]
  Transfer Fcn1 : TransferFcn  Numerator=[1 0]  Denominator=[T_vel 1]
  taum3 : Outport  VectorParamsAs1DForOutWhenUnconnected=off
  wires:
  Transfer Fcn1/1 -> Add/1
  Transfer Fcn/1 -> Add/3
  Sum/1 -> Prop 3/1
  qm3/1 -> Transfer Fcn/1, Sum/2
  Prop 3/1 -> Add/2
  qmd3/1 -> Transfer Fcn1/1, Sum/1
  Gain/1 -> Add1/1
  Add/1 -> Gain1/1, Gain/1
  Integrator/1 -> Add1/2
  Add1/1 -> taum3/1
  Gain1/1 -> Integrator/1

== system limbero_leg_control_DH/Axis Control 2/Axis4  ==
  qmd4 : Inport
  qm4 : Inport  Port=2
  Add : Sum  Inputs=++-
  Add1 : Sum
  Gain : Gain  Gain=kpv(4)
  Gain1 : Gain  Gain=kpv(4)/Tiv
  Integrator : Integrator
  Prop 4 : Gain  Gain=kpp
  Sum : Sum  Inputs=|+-
  Transfer Fcn : TransferFcn  Numerator=[1 0]  Denominator=[T_vel 1]
  Transfer Fcn1 : TransferFcn  Numerator=[1 0]  Denominator=[T_vel 1]
  taum4 : Outport  VectorParamsAs1DForOutWhenUnconnected=off
  wires:
  Transfer Fcn1/1 -> Add/1
  Transfer Fcn/1 -> Add/3
  Sum/1 -> Prop 4/1
  qm4/1 -> Transfer Fcn/1, Sum/2
  Prop 4/1 -> Add/2
  qmd4/1 -> Transfer Fcn1/1, Sum/1
  Gain1/1 -> Integrator/1
  Gain/1 -> Add1/1
  Add/1 -> Gain1/1, Gain/1
  Integrator/1 -> Add1/2
  Add1/1 -> taum4/1

== system limbero_leg_control_DH/Axis Control 2/Axis5  ==
  qmd5 : Inport
  qm5 : Inport  Port=2
  Add : Sum  Inputs=++-
  Add1 : Sum
  Gain : Gain  Gain=kpv(5)
  Gain1 : Gain  Gain=kpv(5)/Tiv
  Integrator : Integrator
  Prop 5 : Gain  Gain=kpp
  Sum : Sum  Inputs=|+-
  Transfer Fcn : TransferFcn  Numerator=[1 0]  Denominator=[T_vel 1]
  Transfer Fcn1 : TransferFcn  Numerator=[1 0]  Denominator=[T_vel 1]
  taum5 : Outport  VectorParamsAs1DForOutWhenUnconnected=off
  wires:
  Transfer Fcn1/1 -> Add/1
  Transfer Fcn/1 -> Add/3
  Sum/1 -> Prop 5/1
  qm5/1 -> Transfer Fcn/1, Sum/2
  Prop 5/1 -> Add/2
  qmd5/1 -> Transfer Fcn1/1, Sum/1
  Gain1/1 -> Integrator/1
  Gain/1 -> Add1/1
  Add/1 -> Gain1/1, Gain/1
  Integrator/1 -> Add1/2
  Add1/1 -> taum5/1

== system limbero_leg_control_DH/Axis Control 2/Axis6  ==
  qmd6 : Inport
  qm6 : Inport  Port=2
  Add : Sum  Inputs=++-
  Add1 : Sum
  Gain : Gain  Gain=kpv(6)
  Gain1 : Gain  Gain=kpv(6)/Tiv
  Integrator : Integrator
  Prop 6 : Gain  Gain=kpp
  Sum : Sum  Inputs=|+-
  Transfer Fcn : TransferFcn  Numerator=[1 0]  Denominator=[T_vel 1]
  Transfer Fcn1 : TransferFcn  Numerator=[1 0]  Denominator=[T_vel 1]
  taum6 : Outport  VectorParamsAs1DForOutWhenUnconnected=off
  wires:
  Transfer Fcn1/1 -> Add/1
  Transfer Fcn/1 -> Add/3
  Sum/1 -> Prop 6/1
  qm6/1 -> Transfer Fcn/1, Sum/2
  Prop 6/1 -> Add/2
  qmd6/1 -> Transfer Fcn1/1, Sum/1
  Gain/1 -> Add1/1
  Add/1 -> Gain1/1, Gain/1
  Integrator/1 -> Add1/2
  Add1/1 -> taum6/1
  Gain1/1 -> Integrator/1

== system limbero_leg_control_DH/Axis Control 2/Axis7  ==
  qmd7 : Inport
  qm7 : Inport  Port=2
  Add : Sum  Inputs=++-
  Add1 : Sum
  Gain : Gain  Gain=kpv(7)
  Gain1 : Gain  Gain=kpv(7)/Tiv
  Integrator : Integrator
  Prop 7 : Gain  Gain=kpp
  Sum : Sum  Inputs=|+-
  Transfer Fcn : TransferFcn  Numerator=[1 0]  Denominator=[T_vel 1]
  Transfer Fcn1 : TransferFcn  Numerator=[1 0]  Denominator=[T_vel 1]
  taum7 : Outport  VectorParamsAs1DForOutWhenUnconnected=off
  wires:
  qmd7/1 -> Transfer Fcn1/1, Sum/1
  Prop 7/1 -> Add/2
  qm7/1 -> Transfer Fcn/1, Sum/2
  Sum/1 -> Prop 7/1
  Transfer Fcn/1 -> Add/3
  Transfer Fcn1/1 -> Add/1
  Gain1/1 -> Integrator/1
  Gain/1 -> Add1/1
  Add/1 -> Gain1/1, Gain/1
  Integrator/1 -> Add1/2
  Add1/1 -> taum7/1

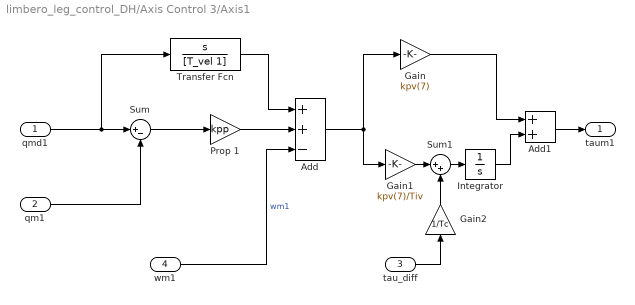
== system limbero_leg_control_DH/Axis Control 3/Axis1  ==
  qmd1 : Inport
  qm1 : Inport  Port=2
  tau_diff : Inport  Port=3
  wm1 : Inport  Port=4
  Add : Sum  Inputs=++-
  Add1 : Sum
  Gain : Gain  Gain=kpv(7)
  Gain1 : Gain  Gain=kpv(7)/Tiv
  Gain2 : Gain  Gain=1/Tc
  Integrator : Integrator
  Prop 1 : Gain  Gain=kpp
  Sum : Sum  Inputs=|+-
  Sum1 : Sum  Inputs=|++
  Transfer Fcn : TransferFcn  Numerator=[1 0]  Denominator=[T_vel 1]
  taum1 : Outport  VectorParamsAs1DForOutWhenUnconnected=off
  wires:
  Transfer Fcn/1 -> Add/1
  Sum/1 -> Prop 1/1
  qm1/1 -> Sum/2
  Prop 1/1 -> Add/2
  Add/1 -> Gain1/1, Gain/1
  qmd1/1 -> Transfer Fcn/1, Sum/1
  Add1/1 -> taum1/1
  Gain/1 -> Add1/1
  Gain1/1 -> Sum1/1
  Sum1/1 -> Integrator/1
  Integrator/1 -> Add1/2
  Gain2/1 -> Sum1/2
  tau_diff/1 -> Gain2/1
  wm1/1 -> Add/3  "wm1"

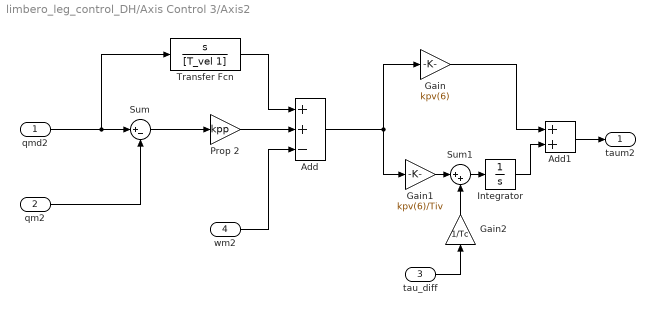
== system limbero_leg_control_DH/Axis Control 3/Axis2  ==
  qmd2 : Inport
  qm2 : Inport  Port=2
  tau_diff : Inport  Port=3
  wm2 : Inport  Port=4
  Add : Sum  Inputs=++-
  Add1 : Sum
  Gain : Gain  Gain=kpv(6)
  Gain1 : Gain  Gain=kpv(6)/Tiv
  Gain2 : Gain  Gain=1/Tc
  Integrator : Integrator
  Prop 2 : Gain  Gain=kpp
  Sum : Sum  Inputs=|+-
  Sum1 : Sum  Inputs=|++
  Transfer Fcn : TransferFcn  Numerator=[1 0]  Denominator=[T_vel 1]
  taum2 : Outport  VectorParamsAs1DForOutWhenUnconnected=off
  wires:
  Transfer Fcn/1 -> Add/1
  Sum/1 -> Prop 2/1
  qm2/1 -> Sum/2
  Prop 2/1 -> Add/2
  qmd2/1 -> Transfer Fcn/1, Sum/1
  Sum1/1 -> Integrator/1
  Gain1/1 -> Sum1/1
  Gain/1 -> Add1/1
  Add/1 -> Gain1/1, Gain/1
  tau_diff/1 -> Gain2/1
  Integrator/1 -> Add1/2
  Add1/1 -> taum2/1
  Gain2/1 -> Sum1/2
  wm2/1 -> Add/3

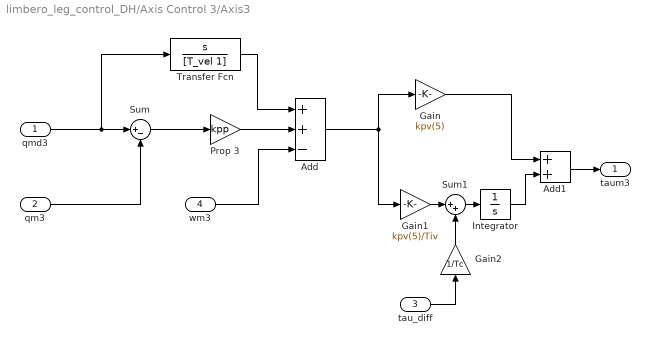
== system limbero_leg_control_DH/Axis Control 3/Axis3  ==
  qmd3 : Inport
  qm3 : Inport  Port=2
  tau_diff : Inport  Port=3
  wm3 : Inport  Port=4
  Add : Sum  Inputs=++-
  Add1 : Sum
  Gain : Gain  Gain=kpv(5)
  Gain1 : Gain  Gain=kpv(5)/Tiv
  Gain2 : Gain  Gain=1/Tc
  Integrator : Integrator
  Prop 3 : Gain  Gain=kpp
  Sum : Sum  Inputs=|+-
  Sum1 : Sum  Inputs=|++
  Transfer Fcn : TransferFcn  Numerator=[1 0]  Denominator=[T_vel 1]
  taum3 : Outport  VectorParamsAs1DForOutWhenUnconnected=off
  wires:
  Transfer Fcn/1 -> Add/1
  wm3/1 -> Add/3
  Sum/1 -> Prop 3/1
  qm3/1 -> Sum/2
  Prop 3/1 -> Add/2
  qmd3/1 -> Transfer Fcn/1, Sum/1
  Sum1/1 -> Integrator/1
  Gain1/1 -> Sum1/1
  Gain/1 -> Add1/1
  Add/1 -> Gain1/1, Gain/1
  tau_diff/1 -> Gain2/1
  Integrator/1 -> Add1/2
  Add1/1 -> taum3/1
  Gain2/1 -> Sum1/2

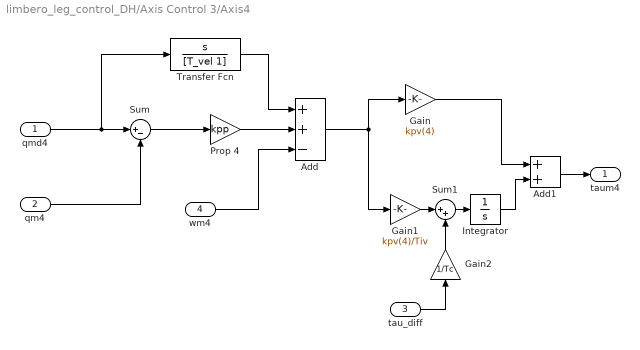
== system limbero_leg_control_DH/Axis Control 3/Axis4  ==
  qmd4 : Inport
  qm4 : Inport  Port=2
  tau_diff : Inport  Port=3
  wm4 : Inport  Port=4
  Add : Sum  Inputs=++-
  Add1 : Sum
  Gain : Gain  Gain=kpv(4)
  Gain1 : Gain  Gain=kpv(4)/Tiv
  Gain2 : Gain  Gain=1/Tc
  Integrator : Integrator
  Prop 4 : Gain  Gain=kpp
  Sum : Sum  Inputs=|+-
  Sum1 : Sum  Inputs=|++
  Transfer Fcn : TransferFcn  Numerator=[1 0]  Denominator=[T_vel 1]
  taum4 : Outport  VectorParamsAs1DForOutWhenUnconnected=off
  wires:
  Transfer Fcn/1 -> Add/1
  wm4/1 -> Add/3
  Sum/1 -> Prop 4/1
  qm4/1 -> Sum/2
  Prop 4/1 -> Add/2
  qmd4/1 -> Transfer Fcn/1, Sum/1
  Sum1/1 -> Integrator/1
  Gain1/1 -> Sum1/1
  Gain/1 -> Add1/1
  Add/1 -> Gain1/1, Gain/1
  tau_diff/1 -> Gain2/1
  Integrator/1 -> Add1/2
  Add1/1 -> taum4/1
  Gain2/1 -> Sum1/2

== system limbero_leg_control_DH/Axis Control 3/Axis5  ==
  qmd5 : Inport
  qm5 : Inport  Port=2
  tau_diff : Inport  Port=3
  wm5 : Inport  Port=4
  Add : Sum  Inputs=++-
  Add1 : Sum
  Gain : Gain  Gain=kpv(3)
  Gain1 : Gain  Gain=kpv(3)/Tiv
  Gain2 : Gain  Gain=1/Tc
  Integrator : Integrator
  Prop 5 : Gain  Gain=kpp
  Sum : Sum  Inputs=|+-
  Sum1 : Sum  Inputs=|++
  Transfer Fcn : TransferFcn  Numerator=[1 0]  Denominator=[T_vel 1]
  taum5 : Outport  VectorParamsAs1DForOutWhenUnconnected=off
  wires:
  Transfer Fcn/1 -> Add/1
  wm5/1 -> Add/3
  Sum/1 -> Prop 5/1
  qm5/1 -> Sum/2
  Prop 5/1 -> Add/2
  qmd5/1 -> Transfer Fcn/1, Sum/1
  Sum1/1 -> Integrator/1
  Gain1/1 -> Sum1/1
  Gain/1 -> Add1/1
  Add/1 -> Gain1/1, Gain/1
  tau_diff/1 -> Gain2/1
  Integrator/1 -> Add1/2
  Add1/1 -> taum5/1
  Gain2/1 -> Sum1/2

== system limbero_leg_control_DH/Axis Control 3/Axis6  ==
  qmd6 : Inport
  qm6 : Inport  Port=2
  tau_diff : Inport  Port=3
  wm6 : Inport  Port=4
  Add : Sum  Inputs=++-
  Add1 : Sum
  Gain : Gain  Gain=kpv(2)
  Gain1 : Gain  Gain=kpv(2)/Tiv
  Gain2 : Gain  Gain=1/Tc
  Integrator : Integrator
  Prop 6 : Gain  Gain=kpp
  Sum : Sum  Inputs=|+-
  Sum1 : Sum  Inputs=|++
  Transfer Fcn : TransferFcn  Numerator=[1 0]  Denominator=[T_vel 1]
  taum6 : Outport  VectorParamsAs1DForOutWhenUnconnected=off
  wires:
  Transfer Fcn/1 -> Add/1
  wm6/1 -> Add/3
  Sum/1 -> Prop 6/1
  qm6/1 -> Sum/2
  Prop 6/1 -> Add/2
  qmd6/1 -> Transfer Fcn/1, Sum/1
  Sum1/1 -> Integrator/1
  Gain1/1 -> Sum1/1
  Gain/1 -> Add1/1
  Add/1 -> Gain1/1, Gain/1
  tau_diff/1 -> Gain2/1
  Integrator/1 -> Add1/2
  Add1/1 -> taum6/1
  Gain2/1 -> Sum1/2

== system limbero_leg_control_DH/Axis Control 3/Axis7  ==
  qmd7 : Inport
  qm7 : Inport  Port=2
  tau_diff : Inport  Port=3
  wm7 : Inport  Port=4
  Add : Sum  Inputs=++-
  Add1 : Sum
  Gain : Gain  Gain=kpv(1)
  Gain1 : Gain  Gain=kpv(1)/Tiv
  Gain2 : Gain  Gain=1/Tc
  Integrator : Integrator
  Prop 7 : Gain  Gain=kpp
  Sum : Sum  Inputs=|+-
  Sum1 : Sum  Inputs=|++
  Transfer Fcn : TransferFcn  Numerator=[1 0]  Denominator=[T_vel 1]
  taum7 : Outport  VectorParamsAs1DForOutWhenUnconnected=off
  wires:
  qmd7/1 -> Transfer Fcn/1, Sum/1
  Prop 7/1 -> Add/2
  qm7/1 -> Sum/2
  Sum/1 -> Prop 7/1
  wm7/1 -> Add/3
  Transfer Fcn/1 -> Add/1
  Sum1/1 -> Integrator/1
  Gain1/1 -> Sum1/1
  Gain/1 -> Add1/1
  Add/1 -> Gain1/1, Gain/1
  tau_diff/1 -> Gain2/1
  Integrator/1 -> Add1/2
  Add1/1 -> taum7/1
  Gain2/1 -> Sum1/2

== system limbero_leg_control_DH/Axis Control 4/Axis1  ==
  qmd1 : Inport
  qm1 : Inport  Port=2
  tau_diff : Inport  Port=3
  wm1 : Inport  Port=4
  Add : Sum  Inputs=++-
  Add1 : Sum
  Gain : Gain  Gain=kpv(1)
  Gain1 : Gain  Gain=kpv(1)/Tiv
  Gain2 : Gain  Gain=1/Tc
  Integrator : Integrator
  Prop 1 : Gain  Gain=kpp
  Sum : Sum  Inputs=|+-
  Sum1 : Sum  Inputs=|++
  Transfer Fcn : TransferFcn  Numerator=[1 0]  Denominator=[T_vel 1]
  taum1 : Outport  VectorParamsAs1DForOutWhenUnconnected=off
  wires:
  Transfer Fcn/1 -> Add/1
  Sum/1 -> Prop 1/1
  qm1/1 -> Sum/2
  Prop 1/1 -> Add/2
  Add/1 -> Gain1/1, Gain/1
  qmd1/1 -> Transfer Fcn/1, Sum/1
  Add1/1 -> taum1/1
  Gain/1 -> Add1/1
  Gain1/1 -> Sum1/1
  Sum1/1 -> Integrator/1
  Integrator/1 -> Add1/2
  Gain2/1 -> Sum1/2
  tau_diff/1 -> Gain2/1
  wm1/1 -> Add/3  "wm1"

== system limbero_leg_control_DH/Axis Control 4/Axis2  ==
  qmd2 : Inport
  qm2 : Inport  Port=2
  tau_diff : Inport  Port=3
  wm2 : Inport  Port=4
  Add : Sum  Inputs=++-
  Add1 : Sum
  Gain : Gain  Gain=kpv(2)
  Gain1 : Gain  Gain=kpv(2)/Tiv
  Gain2 : Gain  Gain=1/Tc
  Integrator : Integrator
  Prop 2 : Gain  Gain=kpp
  Sum : Sum  Inputs=|+-
  Sum1 : Sum  Inputs=|++
  Transfer Fcn : TransferFcn  Numerator=[1 0]  Denominator=[T_vel 1]
  taum2 : Outport  VectorParamsAs1DForOutWhenUnconnected=off
  wires:
  Transfer Fcn/1 -> Add/1
  Sum/1 -> Prop 2/1
  qm2/1 -> Sum/2
  Prop 2/1 -> Add/2
  qmd2/1 -> Transfer Fcn/1, Sum/1
  Sum1/1 -> Integrator/1
  Gain1/1 -> Sum1/1
  Gain/1 -> Add1/1
  Add/1 -> Gain1/1, Gain/1
  tau_diff/1 -> Gain2/1
  Integrator/1 -> Add1/2
  Add1/1 -> taum2/1
  Gain2/1 -> Sum1/2
  wm2/1 -> Add/3

== system limbero_leg_control_DH/Axis Control 4/Axis3  ==
  qmd3 : Inport
  qm3 : Inport  Port=2
  tau_diff : Inport  Port=3
  wm3 : Inport  Port=4
  Add : Sum  Inputs=++-
  Add1 : Sum
  Gain : Gain  Gain=kpv(3)
  Gain1 : Gain  Gain=kpv(3)/Tiv
  Gain2 : Gain  Gain=1/Tc
  Integrator : Integrator
  Prop 3 : Gain  Gain=kpp
  Sum : Sum  Inputs=|+-
  Sum1 : Sum  Inputs=|++
  Transfer Fcn : TransferFcn  Numerator=[1 0]  Denominator=[T_vel 1]
  taum3 : Outport  VectorParamsAs1DForOutWhenUnconnected=off
  wires:
  Transfer Fcn/1 -> Add/1
  wm3/1 -> Add/3
  Sum/1 -> Prop 3/1
  qm3/1 -> Sum/2
  Prop 3/1 -> Add/2
  qmd3/1 -> Transfer Fcn/1, Sum/1
  Sum1/1 -> Integrator/1
  Gain1/1 -> Sum1/1
  Gain/1 -> Add1/1
  Add/1 -> Gain1/1, Gain/1
  tau_diff/1 -> Gain2/1
  Integrator/1 -> Add1/2
  Add1/1 -> taum3/1
  Gain2/1 -> Sum1/2

== system limbero_leg_control_DH/Axis Control 4/Axis4  ==
  qmd4 : Inport
  qm4 : Inport  Port=2
  tau_diff : Inport  Port=3
  wm4 : Inport  Port=4
  Add : Sum  Inputs=++-
  Add1 : Sum
  Gain : Gain  Gain=kpv(4)
  Gain1 : Gain  Gain=kpv(4)/Tiv
  Gain2 : Gain  Gain=1/Tc
  Integrator : Integrator
  Prop 4 : Gain  Gain=kpp
  Sum : Sum  Inputs=|+-
  Sum1 : Sum  Inputs=|++
  Transfer Fcn : TransferFcn  Numerator=[1 0]  Denominator=[T_vel 1]
  taum4 : Outport  VectorParamsAs1DForOutWhenUnconnected=off
  wires:
  Transfer Fcn/1 -> Add/1
  wm4/1 -> Add/3
  Sum/1 -> Prop 4/1
  qm4/1 -> Sum/2
  Prop 4/1 -> Add/2
  qmd4/1 -> Transfer Fcn/1, Sum/1
  Sum1/1 -> Integrator/1
  Gain1/1 -> Sum1/1
  Gain/1 -> Add1/1
  Add/1 -> Gain1/1, Gain/1
  tau_diff/1 -> Gain2/1
  Integrator/1 -> Add1/2
  Add1/1 -> taum4/1
  Gain2/1 -> Sum1/2

== system limbero_leg_control_DH/Axis Control 4/Axis5  ==
  qmd5 : Inport
  qm5 : Inport  Port=2
  tau_diff : Inport  Port=3
  wm5 : Inport  Port=4
  Add : Sum  Inputs=++-
  Add1 : Sum
  Gain : Gain  Gain=kpv(5)
  Gain1 : Gain  Gain=kpv(5)/Tiv
  Gain2 : Gain  Gain=1/Tc
  Integrator : Integrator
  Prop 5 : Gain  Gain=kpp
  Sum : Sum  Inputs=|+-
  Sum1 : Sum  Inputs=|++
  Transfer Fcn : TransferFcn  Numerator=[1 0]  Denominator=[T_vel 1]
  taum5 : Outport  VectorParamsAs1DForOutWhenUnconnected=off
  wires:
  Transfer Fcn/1 -> Add/1
  wm5/1 -> Add/3
  Sum/1 -> Prop 5/1
  qm5/1 -> Sum/2
  Prop 5/1 -> Add/2
  qmd5/1 -> Transfer Fcn/1, Sum/1
  Sum1/1 -> Integrator/1
  Gain1/1 -> Sum1/1
  Gain/1 -> Add1/1
  Add/1 -> Gain1/1, Gain/1
  tau_diff/1 -> Gain2/1
  Integrator/1 -> Add1/2
  Add1/1 -> taum5/1
  Gain2/1 -> Sum1/2

== system limbero_leg_control_DH/Axis Control 4/Axis6  ==
  qmd6 : Inport
  qm6 : Inport  Port=2
  tau_diff : Inport  Port=3
  wm6 : Inport  Port=4
  Add : Sum  Inputs=++-
  Add1 : Sum
  Gain : Gain  Gain=kpv(6)
  Gain1 : Gain  Gain=kpv(6)/Tiv
  Gain2 : Gain  Gain=1/Tc
  Integrator : Integrator
  Prop 6 : Gain  Gain=kpp
  Sum : Sum  Inputs=|+-
  Sum1 : Sum  Inputs=|++
  Transfer Fcn : TransferFcn  Numerator=[1 0]  Denominator=[T_vel 1]
  taum6 : Outport  VectorParamsAs1DForOutWhenUnconnected=off
  wires:
  Transfer Fcn/1 -> Add/1
  wm6/1 -> Add/3
  Sum/1 -> Prop 6/1
  qm6/1 -> Sum/2
  Prop 6/1 -> Add/2
  qmd6/1 -> Transfer Fcn/1, Sum/1
  Sum1/1 -> Integrator/1
  Gain1/1 -> Sum1/1
  Gain/1 -> Add1/1
  Add/1 -> Gain1/1, Gain/1
  tau_diff/1 -> Gain2/1
  Integrator/1 -> Add1/2
  Add1/1 -> taum6/1
  Gain2/1 -> Sum1/2

== system limbero_leg_control_DH/Axis Control 4/Axis7  ==
  qmd7 : Inport
  qm7 : Inport  Port=2
  tau_diff : Inport  Port=3
  wm7 : Inport  Port=4
  Add : Sum  Inputs=++-
  Add1 : Sum
  Gain : Gain  Gain=kpv(7)
  Gain1 : Gain  Gain=kpv(7)/Tiv
  Gain2 : Gain  Gain=1/Tc
  Integrator : Integrator
  Prop 7 : Gain  Gain=kpp
  Sum : Sum  Inputs=|+-
  Sum1 : Sum  Inputs=|++
  Transfer Fcn : TransferFcn  Numerator=[1 0]  Denominator=[T_vel 1]
  taum7 : Outport  VectorParamsAs1DForOutWhenUnconnected=off
  wires:
  qmd7/1 -> Transfer Fcn/1, Sum/1
  Prop 7/1 -> Add/2
  qm7/1 -> Sum/2
  Sum/1 -> Prop 7/1
  wm7/1 -> Add/3
  Transfer Fcn/1 -> Add/1
  Sum1/1 -> Integrator/1
  Gain1/1 -> Sum1/1
  Gain/1 -> Add1/1
  Add/1 -> Gain1/1, Gain/1
  tau_diff/1 -> Gain2/1
  Integrator/1 -> Add1/2
  Add1/1 -> taum7/1
  Gain2/1 -> Sum1/2

== system limbero_leg_control_DH/Joint_Traj Generator/Subsystem ==
  Add : Sum  Inputs=++++
  Add1 : Sum
  Constant : Constant  Value=qz(2)
  Integrator : Integrator
  Integrator1 : Integrator
  Scope : Scope
  Scope1 : Scope
  Scope2 : Scope
  Step : Step  Time=t0  After=q_dotdot(2)  SampleTime=0
  Step1 : Step  Time=t0+t_acc(2)  After=-q_dotdot(2)  SampleTime=0
  Step2 : Step  Time=t0+t_tot-t_acc(2)  After=-q_dotdot(2)  SampleTime=0
  Step3 : Step  Time=t0+t_tot  After=q_dotdot(2)  SampleTime=0
  B2C : Outport
  wires:
  Step3/1 -> Add/4
  Add/1 -> Scope2/1, Integrator/1
  Integrator1/1 -> Add1/2
  Step1/1 -> Add/2
  Step2/1 -> Add/3
  Step/1 -> Add/1
  Integrator/1 -> Scope1/1, Integrator1/1
  Constant/1 -> Add1/1
  Add1/1 -> B2C/1, Scope/1

== system limbero_leg_control_DH/Joint_Traj Generator/Subsystem1 ==
  Add : Sum  Inputs=++++
  Add1 : Sum
  Constant : Constant  Value=qz(3)
  Integrator : Integrator
  Integrator1 : Integrator
  Scope : Scope
  Scope1 : Scope
  Scope2 : Scope
  Step : Step  Time=t0  After=q_dotdot(3)  SampleTime=0
  Step1 : Step  Time=t0+t_acc(3)  After=-q_dotdot(3)  SampleTime=0
  Step2 : Step  Time=t0+t_tot-t_acc(3)  After=-q_dotdot(3)  SampleTime=0
  Step3 : Step  Time=t0+t_tot  After=q_dotdot(3)  SampleTime=0
  C2F : Outport
  wires:
  Add1/1 -> Scope/1, C2F/1
  Constant/1 -> Add1/1
  Integrator/1 -> Integrator1/1, Scope1/1
  Step/1 -> Add/1
  Step2/1 -> Add/3
  Step1/1 -> Add/2
  Integrator1/1 -> Add1/2
  Add/1 -> Integrator/1, Scope2/1
  Step3/1 -> Add/4

== system limbero_leg_control_DH/Joint_Traj Generator1/Subsystem ==
  Add : Sum  Inputs=++++
  Add1 : Sum
  Constant : Constant  Value=qz(2)
  Integrator : Integrator
  Integrator1 : Integrator
  Scope : Scope
  Scope1 : Scope
  Scope2 : Scope
  Step : Step  Time=t0  After=q_dotdot(2)  SampleTime=0
  Step1 : Step  Time=t0+t_acc(2)  After=-q_dotdot(2)  SampleTime=0
  Step2 : Step  Time=t0+t_tot-t_acc(2)  After=-q_dotdot(2)  SampleTime=0
  Step3 : Step  Time=t0+t_tot  After=q_dotdot(2)  SampleTime=0
  B2C : Outport
  wires:
  Step3/1 -> Add/4
  Add/1 -> Scope2/1, Integrator/1
  Integrator1/1 -> Add1/2
  Step1/1 -> Add/2
  Step2/1 -> Add/3
  Step/1 -> Add/1
  Integrator/1 -> Scope1/1, Integrator1/1
  Constant/1 -> Add1/1
  Add1/1 -> B2C/1, Scope/1

== system limbero_leg_control_DH/Joint_Traj Generator1/Subsystem1 ==
  Add : Sum  Inputs=++++
  Add1 : Sum
  Constant : Constant  Value=qz(3)
  Integrator : Integrator
  Integrator1 : Integrator
  Scope : Scope
  Scope1 : Scope
  Scope2 : Scope
  Step : Step  Time=t0  After=q_dotdot(3)  SampleTime=0
  Step1 : Step  Time=t0+t_acc(3)  After=-q_dotdot(3)  SampleTime=0
  Step2 : Step  Time=t0+t_tot-t_acc(3)  After=-q_dotdot(3)  SampleTime=0
  Step3 : Step  Time=t0+t_tot  After=q_dotdot(3)  SampleTime=0
  C2F : Outport
  wires:
  Add1/1 -> Scope/1, C2F/1
  Constant/1 -> Add1/1
  Integrator/1 -> Integrator1/1, Scope1/1
  Step/1 -> Add/1
  Step2/1 -> Add/3
  Step1/1 -> Add/2
  Integrator1/1 -> Add1/2
  Add/1 -> Integrator/1, Scope2/1
  Step3/1 -> Add/4

== matlab function limbero_leg_control_DH/MATLAB Function1 ==
  data: q input; g output; d parameter; a parameter; alpha parameter; offset parameter; r_cm parameter; masses parameter
function g = fcn(q, d, a, alpha, offset, r_cm, masses)
g = Gravity_compensation(a,d,alpha,offset, r_cm, masses, q, 0);

== matlab function limbero_leg_control_DH/MATLAB Function ==
  data: q input; g output; d_contact parameter; a_contact parameter; alpha_contact parameter; offset_contact parameter; r_cm_contact parameter; masses_contact parameter
function g = fcn(q, d_contact, a_contact, alpha_contact, offset_contact, r_cm_contact, masses_contact)
g = Gravity_compensation(a_contact,d_contact,alpha_contact,offset_contact, r_cm_contact, masses_contact, q, 0);

== matlab function limbero_leg_control_DH/MATLAB Function2 ==
  data: q input; g output; d parameter; a parameter; alpha parameter; offset parameter; r_cm parameter; masses parameter
function g = fcn(q, d, a, alpha, offset, r_cm, masses)
g = Gravity_compensation(a,d,alpha,offset, r_cm, masses, q, 0);

== matlab function limbero_leg_control_DH/MATLAB Function3 ==
  data: q input; g output; d parameter; a parameter; alpha parameter; offset parameter; r_cm parameter; masses parameter
function g = fcn(q, d, a, alpha, offset, r_cm, masses)
g = Gravity_compensation(a,d,alpha,offset, r_cm, masses, q, 0);
